simulink model "RIR_Zapocet_Simulink_Vlcek"  (R2019b)
settings: Solver=FixedStepAuto  StartTime=0.0  StopTime=3  FixedStep=1e-3  RelTol=1e-3
values from neighbouring files (symbols this model uses):
  A = [0 1 0 0; -k/m1 -b/m1 k/m1 0; 0 0 0 1; k/m2 0 -k/m2 0]    [RIR_Zapocet_Matlab_Vlcek.m]
  B = [0; 0; 0; 1/m2]    [RIR_Zapocet_Matlab_Vlcek.m]
  C = [1 0 0 0]    [RIR_Zapocet_Matlab_Vlcek.m]
  K = rK(1:4)    [RIR_Zapocet_Matlab_Vlcek.m]
  KI = -rK(5)    [RIR_Zapocet_Matlab_Vlcek.m]
settings Model: Creator=x  LastModifiedBy=x
settings SolverCC: MaxConsecutiveZCs=10000

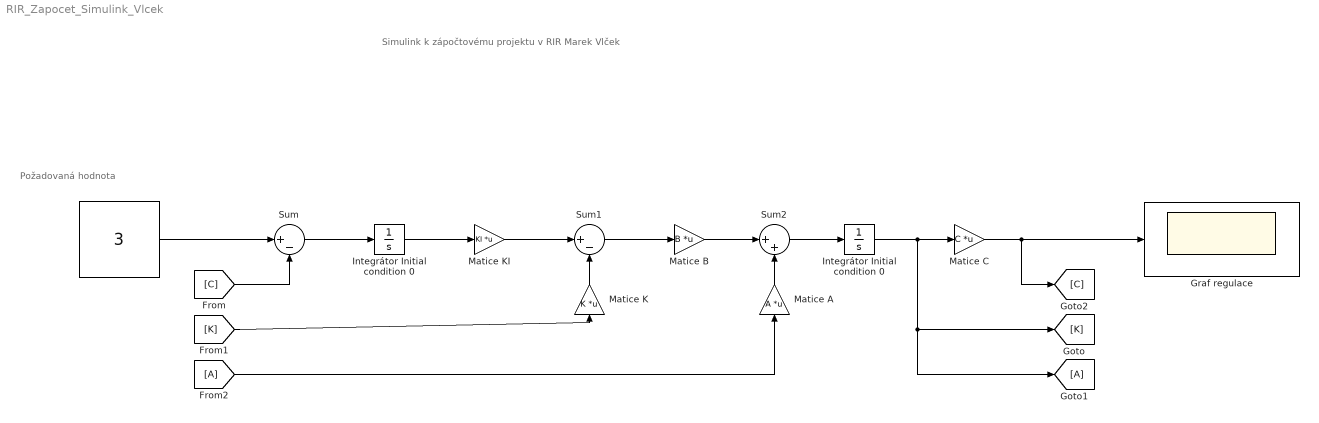
== system RIR_Zapocet_Simulink_Vlcek ==
  note: Simulink k zápočtovému projektu v RIR
      | 										Marek Vlček
  note: Požadovaná hodnota
  " " : Constant  Value=3
  " Matice A" : Gain  Gain=A  Multiplication=Matrix(K*u)
  " Matice K" : Gain  Gain=K  Multiplication=Matrix(K*u)
  "Graf regulace " : Scope
  "Integrátor Initial condition 0 " : Integrator  InitialCondition=0.75
  "Integrátor Initial condition 0 " : Integrator
  Matice B : Gain  Gain=B  Multiplication=Matrix(K*u)
  Matice C : Gain  Gain=C  Multiplication=Matrix(K*u)
  Matice KI : Gain  Gain=KI  Multiplication=Matrix(K*u)
  Sum : Sum  Inputs=|+-
  Sum1 : Sum  Inputs=|+-
  Sum2 : Sum  Inputs=|++
  wires:
  Sum/1 -> "Integrátor Initial condition 0 "/1
  " "/1 -> Sum/1
  Sum1/1 -> Matice B/1
  Matice KI/1 -> Sum1/1
  "Integrátor Initial condition 0 "/1 -> Matice KI/1
  Matice B/1 -> Sum2/1
  Sum2/1 -> "Integrátor Initial condition 0 "/1
  Matice C/1 -> [C], "Graf regulace "/1
  "Integrátor Initial condition 0 "/1 -> [A], [K], Matice C/1
  " Matice A"/1 -> Sum2/2
  " Matice K"/1 -> Sum1/2
  [C] -> Sum/2
  [A] -> " Matice A"/1
  [K] -> " Matice K"/1
